simulink model "SIM_Pgrado_Raul"  (R2017a)
settings: Solver=ode45  StartTime=0.0  StopTime=0.2  RelTol=1e-3  EnableMultiTasking=on
undefined symbols (not defined in the file): st_time, st_time3
libraries: fl_lib x50, nesl_utility x19, powerlib_meascontrol x6, dsparch4 x5
settings Model: Creator=erich  LastModifiedBy=erich
settings DataIOCC: LimitDataPoints=on  SaveFormat=StructureWithTime
settings OptimizationCC: LifeSpan=inf
settings DebuggingCC: SFUnexpectedBacktrackingDiag=warning  SFNoUnconditionalDefaultTransitionDiag=warning  SFExecutionAtInitializationDiag=none
settings HardwareCC: ProdBitPerSizeT=32  ProdBitPerPtrDiffT=32  ProdWordSize=32  ProdHWDeviceType=Specified
settings ModelReferenceCC: PropagateSignalLabelsOutOfModel=off
settings GRTTargetCC: TargetLangStandard=C89/C90 (ANSI)
settings ConfigComp: CovMetricSettings=dw  CovHtmlReporting=on  CovSaveCumulativeToWorkspaceVar=on  CovSaveSingleToWorkspaceVar=on  CovExternalEMLEnable=off

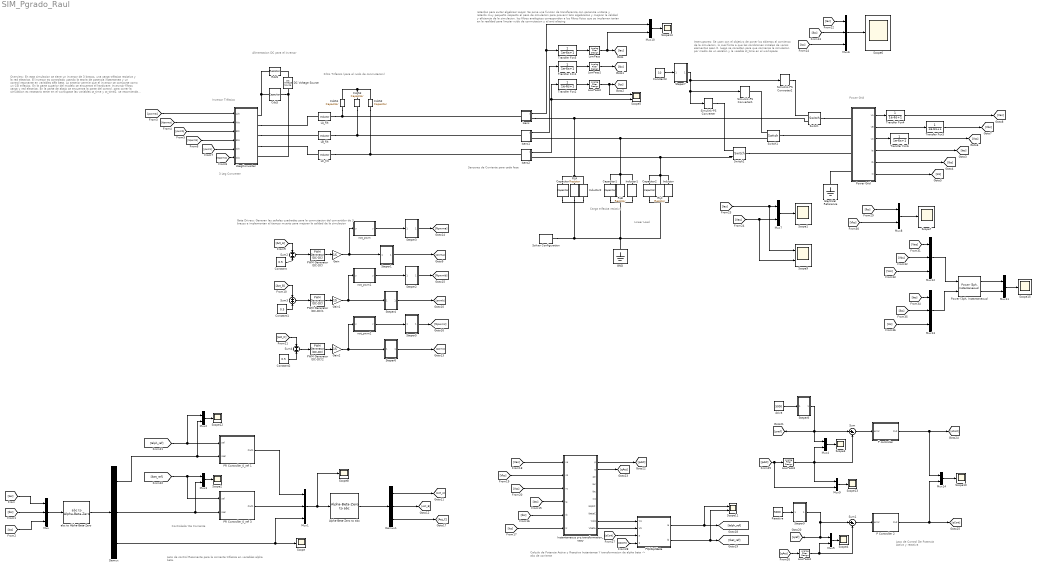
== system SIM_Pgrado_Raul ==
  note: Inversor Trifasico
  note: Overview:
      | En esta simulacion se tiene un inversor
      | de 3 brazos, una carga trifasica resistiva
      | y la red electrica. El inversor es controlado
      | usando la teoria de potencia instantanea
      | y un control resonante en variables alfa beta.
      | Lo anterior permie que el inversor se comporte
      | como un CSI trifasico.
      |
      | En la parte superior del modelo se encuentra el hardware:
      | Invevrsor filtros carga y red electrica.
      |
      | En la parte de abajo se encuentra la parte del control.
      |
      | para correr la simulacion es necesario tener en el workspace
      | las variables st_time y st_time2. se recomienda 10ms y 20 ms
      | respectivamente.
  note: Lazo de Control De
      | Potencia Activa y reactiva
  note: Calculo de Potencia Activa y Reactiva Instantanea
      | Y transformacion de alpha beta -> abc de corriente
  note: retardos para evitar algebraic Loops:
      | Se pone una funcion de transferencia con ganancia unitaria
      | y retardo muy pequeño respecto al paso de simulacion para prevenir
      | lazo algebraicos y mejorar la calidad y eficiencia de la simulacion.
      | los filtros analogicos corresponden a los filtros fisico que se implemen
      | tarian en la realidad para limpiar ruido de conmutacion y el anti aliasing
  note: Power Grid
  note: Linear Load
  note: 3 Leg Converter
  note: Controlador De Corriente
  note: Alimentacion DC
      | para el inversor
  note: Filtro Trifasico
      | (para el ruido de conmutacion)
  note: Sensores de Corriente para cada fase
  note: Carga trifasica resistiva
  note: Interruptores:
      | Se usan con el objetivo de poner
      | los abiertos al comienzo de la simulacion,
      | lo cual forza a que las condiciones iniciales
      | de varios elementos sean 0. luego se conectan
      | para que comience la simulacion por medio de
      | un escalon y la vaiable st_time en el workspace
  note: Lazo de control Resonante para la
      | corriente trifasica en variables alpha beta.
  note: Gate Drivers: Generan las señales cuadradas para
      | la conmutacion del convertidor de 3 brazos e implementan el
      | tiempo muerto para mejorar la calidad de la simulacion
  3LegConverter : Subsystem
  Aciva : Constant  Value=5000
  Alpha-Beta-Zero to abc : powerlib_meascontrol/Transformations/Alpha-Beta-Zero to abc
      settings: SourceProductName=Simscape Power Systems  SourceProductBaseCode=PS
  Capacitor : fl_lib/Electrical/Electrical Elements/Capacitor  c=100e-6 uF  r=1e-6 Ohm  g=0 1/Ohm  i_specify=off  i_priority=None  i=0 A  i_nominal_specify=off  i_nominal_unit=A  i_nominal_value=1  v_specify=off  v_priority=None  v=0 V  v_nominal_specify=off  v_nominal_unit=V  v_nominal_value=1  vc_specify=off  vc_priority=High  vc=0 V  vc_nominal_specify=off  vc_nominal_unit=V  vc_nominal_value=1
  Capacitor1 : fl_lib/Electrical/Electrical Elements/Capacitor  c=100e-6 uF  r=1e-6 Ohm  g=0 1/Ohm  i_specify=off  i_priority=None  i=0 A  i_nominal_specify=off  i_nominal_unit=A  i_nominal_value=1  v_specify=off  v_priority=None  v=0 V  v_nominal_specify=off  v_nominal_unit=V  v_nominal_value=1  vc_specify=off  vc_priority=High  vc=0 V  vc_nominal_specify=off  vc_nominal_unit=V  vc_nominal_value=1
  Capacitor2 : fl_lib/Electrical/Electrical Elements/Capacitor  c=100e-6 uF  r=1e-6 Ohm  g=0 1/Ohm  i_specify=off  i_priority=None  i=0 A  i_nominal_specify=off  i_nominal_unit=A  i_nominal_value=1  v_specify=off  v_priority=None  v=0 V  v_nominal_specify=off  v_nominal_unit=V  v_nominal_value=1  vc_specify=off  vc_priority=High  vc=0 V  vc_nominal_specify=off  vc_nominal_unit=V  vc_nominal_value=1
  CdcS : fl_lib/Electrical/Electrical Elements/Capacitor  c=1 uF  r=1e-6 Ohm  g=0 1/Ohm  i_specify=off  i_priority=None  i=0 A  i_nominal_specify=off  i_nominal_unit=A  i_nominal_value=1  v_specify=off  v_priority=None  v=0 V  v_nominal_specify=off  v_nominal_unit=V  v_nominal_value=1  vc_specify=on  vc_priority=High  vc=0 V  vc_nominal_specify=off  vc_nominal_unit=V  vc_nominal_value=1
  CdcS1 : fl_lib/Electrical/Electrical Elements/Capacitor  c=3.5 uF  r=1e-6 Ohm  g=0 1/Ohm  i_specify=off  i_priority=None  i=0 A  i_nominal_specify=off  i_nominal_unit=A  i_nominal_value=1  v_specify=off  v_priority=None  v=0 V  v_nominal_specify=off  v_nominal_unit=V  v_nominal_value=1  vc_specify=on  vc_priority=High  vc=0 V  vc_nominal_specify=off  vc_nominal_unit=V  vc_nominal_value=1
  CdcS2 : fl_lib/Electrical/Electrical Elements/Capacitor  c=3.5 uF  r=1e-6 Ohm  g=0 1/Ohm  i_specify=off  i_priority=None  i=0 A  i_nominal_specify=off  i_nominal_unit=A  i_nominal_value=1  v_specify=off  v_priority=None  v=0 V  v_nominal_specify=off  v_nominal_unit=V  v_nominal_value=1  vc_specify=on  vc_priority=High  vc=0 V  vc_nominal_specify=off  vc_nominal_unit=V  vc_nominal_value=1
  CdcS3 : fl_lib/Electrical/Electrical Elements/Capacitor  c=3.5 uF  r=1e-6 Ohm  g=0 1/Ohm  i_specify=off  i_priority=None  i=0 A  i_nominal_specify=off  i_nominal_unit=A  i_nominal_value=1  v_specify=off  v_priority=None  v=0 V  v_nominal_specify=off  v_nominal_unit=V  v_nominal_value=1  vc_specify=on  vc_priority=High  vc=0 V  vc_nominal_specify=off  vc_nominal_unit=V  vc_nominal_value=1
  Constant : Constant  Value=0.5
  Constant1 : Constant  Value=0.5
  Constant2 : Constant  Value=0.5
  Constant3 : Constant  Value=10
  DC Voltage Source : fl_lib/Electrical/Electrical Sources/DC Voltage Source  v0=420 V
  Demux : Demux  Outputs=3
  Demux1 : Demux  Outputs=3
  Electrical Reference : fl_lib/Electrical/Electrical Elements/Electrical Reference
  GND : fl_lib/Electrical/Electrical Elements/Electrical Reference
  Gain : Gain  Gain=15
  Gain1 : Gain  Gain=15
  Gain2 : Gain  Gain=15
  Inductor : fl_lib/Electrical/Electrical Elements/Inductor  l=5200 mH  r=0 Ohm  g=100e-9 1/Ohm  i_specify=off  i_priority=None  i=0 A  i_nominal_specify=off  i_nominal_unit=A  i_nominal_value=1  v_specify=off  v_priority=None  v=0 V  v_nominal_specify=off  v_nominal_unit=V  v_nominal_value=1  i_L_specify=off  i_L_priority=High  i_L=0 A  i_L_nominal_specify=off  i_L_nominal_unit=A  i_L_nominal_value=1
  Inductor1 : fl_lib/Electrical/Electrical Elements/Inductor  l=5200 mH  r=0 Ohm  g=100e-9 1/Ohm  i_specify=off  i_priority=None  i=0 A  i_nominal_specify=off  i_nominal_unit=A  i_nominal_value=1  v_specify=off  v_priority=None  v=0 V  v_nominal_specify=off  v_nominal_unit=V  v_nominal_value=1  i_L_specify=off  i_L_priority=High  i_L=0 A  i_L_nominal_specify=off  i_L_nominal_unit=A  i_L_nominal_value=1
  Inductor2 : fl_lib/Electrical/Electrical Elements/Inductor  l=5200 mH  r=0 Ohm  g=100e-9 1/Ohm  i_specify=off  i_priority=None  i=0 A  i_nominal_specify=off  i_nominal_unit=A  i_nominal_value=1  v_specify=off  v_priority=None  v=0 V  v_nominal_specify=off  v_nominal_unit=V  v_nominal_value=1  i_L_specify=off  i_L_priority=High  i_L=0 A  i_L_nominal_specify=off  i_L_nominal_unit=A  i_L_nominal_value=1
  Instantaneous p-q transformation_copy : MATLAB Function  TreatAsAtomicUnit=on
  Isens : Subsystem
  Isens1 : Subsystem
  Isens2 : Subsystem
  LA_filt : fl_lib/Electrical/Electrical Elements/Inductor  l=6.2 mH  r=0.1 Ohm  g=1e-6 1/Ohm  i_specify=off  i_priority=None  i=0 A  i_nominal_specify=off  i_nominal_unit=A  i_nominal_value=1  v_specify=off  v_priority=None  v=0 V  v_nominal_specify=off  v_nominal_unit=V  v_nominal_value=1  i_L_specify=on  i_L_priority=High  i_L=0 A  i_L_nominal_specify=off  i_L_nominal_unit=A  i_L_nominal_value=1
  LB_filt : fl_lib/Electrical/Electrical Elements/Inductor  l=6.2 mH  r=2 Ohm  g=1e-6 1/Ohm  i_specify=off  i_priority=None  i=0 A  i_nominal_specify=off  i_nominal_unit=A  i_nominal_value=1  v_specify=off  v_priority=None  v=0 V  v_nominal_specify=off  v_nominal_unit=V  v_nominal_value=1  i_L_specify=on  i_L_priority=High  i_L=0 A  i_L_nominal_specify=off  i_L_nominal_unit=A  i_L_nominal_value=1
  LC_filt : fl_lib/Electrical/Electrical Elements/Inductor  l=6.2 mH  r=2 Ohm  g=1e-6 1/Ohm  i_specify=off  i_priority=None  i=0 A  i_nominal_specify=off  i_nominal_unit=A  i_nominal_value=1  v_specify=off  v_priority=None  v=0 V  v_nominal_specify=off  v_nominal_unit=V  v_nominal_value=1  i_L_specify=on  i_L_priority=High  i_L=0 A  i_L_nominal_specify=off  i_L_nominal_unit=A  i_L_nominal_value=1
  LowPass{,1..4} (5 alike) : dsparch4/Analog Filter Design  method=Bessel  filttype=Lowpass  N=1  Wlo=2500*2*pi  Whi=80  Rp=2  Rs=40
  Mux{,1,6,12..13} (5 alike) : Mux  Inputs=3
  Mux{2..5,7..11,14} (10 alike) : Mux  Inputs=2
  "P Controller 2 " : Subsystem
  P controller : Subsystem
  PQ2AlphBeta : MATLAB Function  TreatAsAtomicUnit=on
  PR Controller_0_ref 1 : Subsystem
      mask Display:
      | port_label('input',1,'ref')
      | port_label('input',2,'sens')
      | port_label('output',1,'out')
      | 
      | plot(.4+[0:.01:pi/10], .32+sin(40*[0:.01:pi/10])/13)
      | 
      | plot([.4 .6],.05+[.5 .7])
      | plot([.4 .6],.05+[.9 .7])
      | plot([.4 .4],.05+[.9 .5])
      | 
      | text(.27,.37,'\fontsize{25} \int', 'texmode', 'on')
  PR Controller_0_ref 3 : Subsystem
      mask Display:
      | port_label('input',1,'ref')
      | port_label('input',2,'sens')
      | port_label('output',1,'out')
      | 
      | plot(.4+[0:.01:pi/10], .32+sin(40*[0:.01:pi/10])/13)
      | 
      | plot([.4 .6],.05+[.5 .7])
      | plot([.4 .6],.05+[.9 .7])
      | plot([.4 .4],.05+[.9 .5])
      | 
      | text(.27,.37,'\fontsize{25} \int', 'texmode', 'on')
  PWM Generator (DC-DC) : powerlib_meascontrol/Pulse & Signal Generators/PWM Generator (DC-DC)  Fsw=5000  Ts=0
  PWM Generator (DC-DC)1 : powerlib_meascontrol/Pulse & Signal Generators/PWM Generator (DC-DC)  Fsw=5000  Ts=0
  PWM Generator (DC-DC)2 : powerlib_meascontrol/Pulse & Signal Generators/PWM Generator (DC-DC)  Fsw=5000  Ts=0
  "Power (3ph, Instantaneous)" : powerlib_meascontrol/Measurements/Power (3ph, Instantaneous)
      settings: SourceProductName=Simscape Power Systems
  Power Grid : Subsystem
  RLA : fl_lib/Electrical/Electrical Elements/Resistor  R=15 Ohm  i_specify=off  i_priority=None  i=0 A  i_nominal_specify=off  i_nominal_unit=A  i_nominal_value=1  v_specify=off  v_priority=None  v=0 V  v_nominal_specify=off  v_nominal_unit=V  v_nominal_value=1
  RLB : fl_lib/Electrical/Electrical Elements/Resistor  R=15 Ohm  i_specify=off  i_priority=None  i=0 A  i_nominal_specify=off  i_nominal_unit=A  i_nominal_value=1  v_specify=off  v_priority=None  v=0 V  v_nominal_specify=off  v_nominal_unit=V  v_nominal_value=1
  RLC : fl_lib/Electrical/Electrical Elements/Resistor  R=15 Ohm  i_specify=off  i_priority=None  i=0 A  i_nominal_specify=off  i_nominal_unit=A  i_nominal_value=1  v_specify=off  v_priority=None  v=0 V  v_nominal_specify=off  v_nominal_unit=V  v_nominal_value=1
  RdcS : fl_lib/Electrical/Electrical Elements/Resistor  R=0.1 Ohm  i_specify=off  i_priority=None  i=0 A  i_nominal_specify=off  i_nominal_unit=A  i_nominal_value=1  v_specify=off  v_priority=None  v=0 V  v_nominal_specify=off  v_nominal_unit=V  v_nominal_value=1
  Reactiva : Constant  Value=5000
  Scope{,1..4,6..8,10,12..15} (13 alike) : Scope
  Scope11 : Scope  NumInputPorts=2
  Scope5 : Scope  NumInputPorts=2
  Scope9 : Scope  NumInputPorts=2
  Simulink-PS Converter : nesl_utility/Simulink-PS Converter  PhysicalDomain=network_engine_domain  SubClassName=ps_input  LeftPortType=input  RightPortType=output  PseudoPeriodic=off  Frequencies=[]  NoiseDistribution=none  NoiseParameters=[]  Unit=1  AffineConversion=off  FilteringAndDerivatives=zero  SimscapeFilterOrder=1  InputFilterTimeConstant=0.001  UdotUserProvided=1
  Simulink-PS Converter1 : nesl_utility/Simulink-PS Converter  PhysicalDomain=network_engine_domain  SubClassName=ps_input  LeftPortType=input  RightPortType=output  PseudoPeriodic=off  Frequencies=[]  NoiseDistribution=none  NoiseParameters=[]  Unit=1  AffineConversion=off  FilteringAndDerivatives=zero  SimscapeFilterOrder=1  InputFilterTimeConstant=0.001  UdotUserProvided=1
  Simulink-PS Converter2 : nesl_utility/Simulink-PS Converter  PhysicalDomain=network_engine_domain  SubClassName=ps_input  LeftPortType=input  RightPortType=output  PseudoPeriodic=off  Frequencies=[]  NoiseDistribution=none  NoiseParameters=[]  Unit=1  AffineConversion=off  FilteringAndDerivatives=zero  SimscapeFilterOrder=1  InputFilterTimeConstant=0.001  UdotUserProvided=1
  Solver Configuration : nesl_utility/Solver Configuration  PhysicalDomain=network_engine_domain  SubClassName=solver  LeftPortType=input  RightPortType=generic  Accelerate=off  Tones=[]  Harmonics=[]  SimulateNoise=off  Profile=off  UseLocalSampling=off  EnableSwitchedLinearOptims=on  FrequencyDomain=off  UseCCode=off  RelTol=0.001  AbsTol=1e-06  MinStep=1e-09  ToWorkspace=off  RevertToSquareIcSolve=off  NumHomotopyIterations=100  PhasorMode=off  PhasorModeNumHarmonics=1  OverrideAbsTol=off  DoDC=off  ResidualTolerance=1e-09  UseLocalSolver=on  LocalSolverChoice=NE_BACKWARD_EULER_ADVANCER  LocalSolverSampleTime=1e-6  DoFixedCost=on  MaxNonlinIter=3  MaxModeIter=2  LinearAlgebra=Sparse  DelaysMemoryBudget=1024  AutomaticFiltering=on  FilteringTimeConstant=0.001
  Steper1 : Subsystem
  Steper2 : Subsystem
  Steper3 : Subsystem
  Steper4 : Subsystem
  Steper5 : Subsystem
  Steper6 : Subsystem
  Steper7 : Subsystem
  Steper8 : Subsystem
  Steper9 : Subsystem
  Sum : Sum  Inputs=|+-
  Sum1 : Sum  Inputs=|+-
  Sum2 : Sum
  Sum3 : Sum
  Sum4 : Sum
  Switch : fl_lib/Electrical/Electrical Elements/Switch  R_closed=1 Ohm  G_open=1e-4 1/Ohm  Threshold=4  i_specify=off  i_priority=None  i=0 A  i_nominal_specify=off  i_nominal_unit=A  i_nominal_value=1  v_specify=off  v_priority=None  v=0 V  v_nominal_specify=off  v_nominal_unit=V  v_nominal_value=1
      settings: SourceProductName=Simscape
  Switch1 : fl_lib/Electrical/Electrical Elements/Switch  R_closed=1 Ohm  G_open=1e-4 1/Ohm  Threshold=4  i_specify=off  i_priority=None  i=0 A  i_nominal_specify=off  i_nominal_unit=A  i_nominal_value=1  v_specify=off  v_priority=None  v=0 V  v_nominal_specify=off  v_nominal_unit=V  v_nominal_value=1
      settings: SourceProductName=Simscape
  Switch2 : fl_lib/Electrical/Electrical Elements/Switch  R_closed=1 Ohm  G_open=1e-4 1/Ohm  Threshold=4  i_specify=off  i_priority=None  i=0 A  i_nominal_specify=off  i_nominal_unit=A  i_nominal_value=1  v_specify=off  v_priority=None  v=0 V  v_nominal_specify=off  v_nominal_unit=V  v_nominal_value=1
      settings: SourceProductName=Simscape
  Transfer Fcn{1..6} (6 alike) : TransferFcn  Denominator=[1e-6 1]
  abc to Alpha-Beta-Zero : powerlib_meascontrol/Transformations/abc to Alpha-Beta-Zero
      settings: SourceProductName=Simscape Power Systems
  not_pwm : MATLAB Function  TreatAsAtomicUnit=on
  not_pwm1 : MATLAB Function  TreatAsAtomicUnit=on
  not_pwm2 : MATLAB Function  TreatAsAtomicUnit=on
  wires:
  Mux/1 -> abc to Alpha-Beta-Zero/1
  Isens2/1(i) -> Scope5/2, Transfer Fcn2/1
  Isens1/1(i) -> Transfer Fcn1/1
  [Iac] -> Mux/1
  [Ibc] -> Mux/2
  [Icc] -> Mux/3
  abc to Alpha-Beta-Zero/1 -> Demux/1
  Mux1/1 -> Scope8/1, Alpha-Beta-Zero to abc/1
  PR Controller_0_ref 3/1(Out1) -> Mux1/2
  Alpha-Beta-Zero to abc/1 -> Demux1/1
  [pwma] -> 3LegConverter/1(Ahi)
  [Npwmc] -> 3LegConverter/6(Clo)
  [pwmc] -> 3LegConverter/5(Chi)
  [Npwmb] -> 3LegConverter/4(Blo)
  [pwmb] -> 3LegConverter/3(Bhi)
  [Npwma] -> 3LegConverter/2(Alo)
  PWM Generator (DC-DC)/1 -> Gain/1
  PWM Generator (DC-DC)1/1 -> Gain1/1
  PWM Generator (DC-DC)2/1 -> Gain2/1
  not_pwm/1(y) -> Steper3/1(In1)
  not_pwm1/1(y) -> Steper2/1(In1)
  not_pwm2/1(y) -> Steper5/1(In1)
  Gain/1 -> Steper1/1(In1), not_pwm/1(u)
  Gain1/1 -> Steper4/1(In1), not_pwm1/1(u)
  Gain2/1 -> Steper6/1(In1), not_pwm2/1(u)
  Steper3/1(Out1) -> [Npwma]
  Steper2/1(Out1) -> [Npwmb]
  Steper5/1(Out1) -> [Npwmc]
  Steper4/1(Out1) -> [pwmb]
  Steper6/1(Out1) -> [pwmc]
  Transfer Fcn5/1 -> LowPass/1
  Transfer Fcn1/1 -> LowPass1/1
  Transfer Fcn2/1 -> LowPass2/1
  Demux1/1 -> [Act_A]
  Demux1/2 -> [Act_B]
  Demux1/3 -> [Act_C]
  Demux/1 -> PR Controller_0_ref 1/2(real), Mux2/2
  Demux/2 -> PR Controller_0_ref 3/2(real), Mux3/2
  Aciva/1 -> Steper8/1(In1)
  Power Grid/1(vA) -> Transfer Fcn4/1
  Power Grid/2(vB) -> Transfer Fcn3/1
  Power Grid/3(vC) -> Transfer Fcn6/1
  Power Grid/4(Ia) -> [Ias]
  Power Grid/5(Ib) -> [Ibs]
  Power Grid/6(Ic) -> [Ics]
  Reactiva/1 -> Steper9/1(In1)
  [pCont] -> PQ2AlphBeta/3(p)
  [qCont] -> PQ2AlphBeta/4(q)
  P controller/1(Out) -> Mux14/1, [pCont]
  "P Controller 2 "/1(Out) -> Mux14/2, [qCont]
  Constant/1 -> Sum2/2
  Constant1/1 -> Sum3/2
  Constant2/1 -> Sum4/2
  Sum2/1 -> PWM Generator (DC-DC)/1
  [Act_A] -> Sum2/1
  Sum3/1 -> PWM Generator (DC-DC)1/1
  [Act_B] -> Sum3/1
  Sum4/1 -> PWM Generator (DC-DC)2/1
  [Act_C] -> Sum4/1
  Steper7/1(Out1) -> Simulink-PS Converter/1, Simulink-PS Converter1/1, Simulink-PS Converter2/1
  Constant3/1 -> Steper7/1(In1)
  PR Controller_0_ref 1/1(Out1) -> Mux1/1
  Demux/3 -> Mux1/3, Scope/1
  Instantaneous p-q transformation_copy/2(q) -> [qAct]
  Instantaneous p-q transformation_copy/1(p) -> [pAct]
  Instantaneous p-q transformation_copy/10(VbetA) -> PQ2AlphBeta/2(Vb)
  Instantaneous p-q transformation_copy/9(ValA) -> PQ2AlphBeta/1(Va)
  [Iac] -> Instantaneous p-q transformation_copy/4(ia)
  [Ibc] -> Instantaneous p-q transformation_copy/5(ib)
  [Icc] -> Instantaneous p-q transformation_copy/6(ic)
  [Vcs] -> Instantaneous p-q transformation_copy/3(vc)
  [Vbs] -> Instantaneous p-q transformation_copy/2(vb)
  [Vas] -> Instantaneous p-q transformation_copy/1(va)
  Transfer Fcn4/1 -> [Vas]
  Transfer Fcn3/1 -> [Vbs]
  Transfer Fcn6/1 -> [Vcs]
  [Ialph_ref] -> PR Controller_0_ref 1/1(ref), Mux2/1
  [Ibet_ref] -> PR Controller_0_ref 3/1(ref), Mux3/1
  [qAct] -> LowPass4/1
  Sum/1 -> P controller/1(error)
  Sum1/1 -> "P Controller 2 "/1(error)
  Mux2/1 -> Scope12/1
  Mux3/1 -> Scope2/1
  Mux4/1 -> Scope3/1
  Mux5/1 -> Scope4/1
  Mux6/1 -> Scope6/1
  [Iac] -> Mux6/1
  [Ibc] -> Mux6/2
  [Icc] -> Mux6/3
  [Ias] -> Scope9/1, Mux7/1
  Mux7/1 -> Scope1/1
  [Vas] -> Scope9/2, Mux7/2
  Mux8/1 -> Scope7/1
  [Ibs] -> Mux8/1
  [Vbs] -> Mux8/2
  LowPass/1 -> Mux10/2, [Iac]
  LowPass1/1 -> [Ibc]
  LowPass2/1 -> Scope5/1, [Icc]
  Mux9/1 -> Scope13/1
  Mux10/1 -> Scope14/1
  Isens/1(i) -> Transfer Fcn5/1, Mux10/1
  PQ2AlphBeta/1(Ia) -> [Ialph_ref], Scope11/1
  PQ2AlphBeta/2(Ib) -> [Ibet_ref], Scope11/2
  LowPass3/1 -> Mux9/1, Sum/2, Mux4/2
  LowPass4/1 -> Mux5/2, Sum1/2
  [pAct] -> Mux9/2, LowPass3/1
  Mux11/1 -> Scope15/1
  "Power (3ph, Instantaneous)"/1 -> Mux11/1
  "Power (3ph, Instantaneous)"/2 -> Mux11/2
  [Vas] -> Mux12/1
  [Vbs] -> Mux12/2
  [Vcs] -> Mux12/3
  Mux12/1 -> "Power (3ph, Instantaneous)"/1
  [Ias] -> Mux13/1
  [Ibs] -> Mux13/2
  [Ics] -> Mux13/3
  Mux13/1 -> "Power (3ph, Instantaneous)"/2
  Mux14/1 -> Scope10/1
  Steper1/1(Out1) -> [pwma]
  Steper8/1(Out1) -> Mux4/1, Sum/1, [pref]
  Steper9/1(Out1) -> Sum1/1, Mux5/1, [qref]
  connections:
  Power Grid/LConn4 -- Electrical Reference/LConn1
  Isens/RConn1 -- Switch/RConn2 -- Inductor2/LConn1 -- Capacitor/LConn1 -- RLA/LConn1
  RLC/LConn1 -- Capacitor2/LConn1 -- Inductor/LConn1 -- Isens2/RConn1 -- Switch2/RConn2
  RLB/LConn1 -- Capacitor1/LConn1 -- Inductor1/LConn1 -- Isens1/RConn1 -- Switch1/RConn2
  3LegConverter/RConn2 -- LA_filt/LConn1
  3LegConverter/RConn3 -- LB_filt/LConn1
  3LegConverter/RConn4 -- LC_filt/LConn1
  3LegConverter/RConn1 -- RdcS/LConn1 -- CdcS/LConn1
  DC Voltage Source/RConn1 -- CdcS/RConn1 -- 3LegConverter/RConn5
  Solver Configuration/RConn1 -- Inductor2/RConn1 -- Capacitor/RConn1 -- RLA/RConn1 -- Capacitor2/RConn1 -- Inductor/RConn1 -- RLC/RConn1 -- Capacitor1/RConn1 -- Inductor1/RConn1 -- RLB/RConn1 -- GND/LConn1
  DC Voltage Source/LConn1 -- RdcS/RConn1
  Switch/LConn1 -- Power Grid/LConn1
  Switch1/LConn1 -- Power Grid/LConn2
  Switch2/LConn1 -- Power Grid/LConn3
  Switch1/RConn1 -- Simulink-PS Converter1/RConn1
  Simulink-PS Converter2/RConn1 -- Switch/RConn1
  Simulink-PS Converter/RConn1 -- Switch2/RConn1
  LA_filt/RConn1 -- Isens/LConn1 -- CdcS1/RConn1
  LB_filt/RConn1 -- Isens1/LConn1 -- CdcS3/RConn1
  LC_filt/RConn1 -- Isens2/LConn1 -- CdcS2/RConn1
  CdcS1/LConn1 -- CdcS3/LConn1 -- CdcS2/LConn1

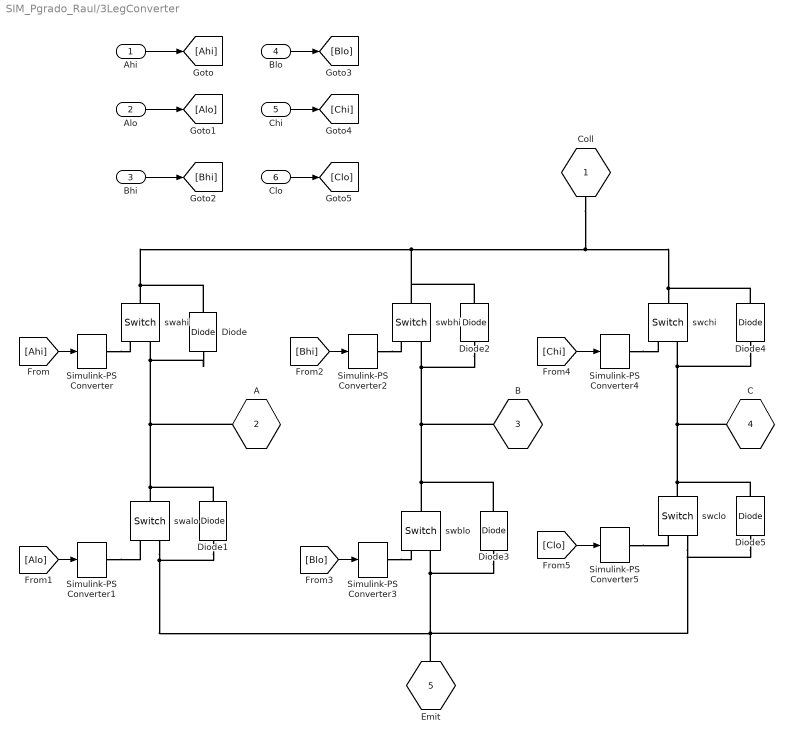
== system SIM_Pgrado_Raul/3LegConverter ==
  Ahi : Inport
  Alo : Inport  Port=2
  Bhi : Inport  Port=3
  Blo : Inport  Port=4
  Chi : Inport  Port=5
  Clo : Inport  Port=6
  Diode{,1..5} (6 alike) : fl_lib/Electrical/Electrical Elements/Diode  Vf=0.6 V  Ron=0.3 Ohm  Goff=1e-8 1/Ohm  i_specify=off  i_priority=None  i=0 A  i_nominal_specify=off  i_nominal_unit=A  i_nominal_value=1  v_specify=off  v_priority=None  v=0 V  v_nominal_specify=off  v_nominal_unit=V  v_nominal_value=1
  Simulink-PS Converter{,1..5} (6 alike) : nesl_utility/Simulink-PS Converter  PhysicalDomain=network_engine_domain  SubClassName=ps_input  LeftPortType=input  RightPortType=output  PseudoPeriodic=off  Frequencies=[]  NoiseDistribution=none  NoiseParameters=[]  Unit=1  AffineConversion=off  FilteringAndDerivatives=zero  SimscapeFilterOrder=1  InputFilterTimeConstant=0.001  UdotUserProvided=1
  swahi : fl_lib/Electrical/Electrical Elements/Switch  R_closed=0.01 Ohm  G_open=1e-8 1/Ohm  Threshold=2  i_specify=off  i_priority=None  i=0 A  i_nominal_specify=off  i_nominal_unit=A  i_nominal_value=1  v_specify=off  v_priority=None  v=0 V  v_nominal_specify=off  v_nominal_unit=V  v_nominal_value=1
      settings: SourceProductName=Simscape
  swalo : fl_lib/Electrical/Electrical Elements/Switch  R_closed=0.01 Ohm  G_open=1e-8 1/Ohm  Threshold=2  i_specify=off  i_priority=None  i=0 A  i_nominal_specify=off  i_nominal_unit=A  i_nominal_value=1  v_specify=off  v_priority=None  v=0 V  v_nominal_specify=off  v_nominal_unit=V  v_nominal_value=1
      settings: SourceProductName=Simscape
  swbhi : fl_lib/Electrical/Electrical Elements/Switch  R_closed=0.01 Ohm  G_open=1e-8 1/Ohm  Threshold=2  i_specify=off  i_priority=None  i=0 A  i_nominal_specify=off  i_nominal_unit=A  i_nominal_value=1  v_specify=off  v_priority=None  v=0 V  v_nominal_specify=off  v_nominal_unit=V  v_nominal_value=1
      settings: SourceProductName=Simscape
  swblo : fl_lib/Electrical/Electrical Elements/Switch  R_closed=0.01 Ohm  G_open=1e-8 1/Ohm  Threshold=2  i_specify=off  i_priority=None  i=0 A  i_nominal_specify=off  i_nominal_unit=A  i_nominal_value=1  v_specify=off  v_priority=None  v=0 V  v_nominal_specify=off  v_nominal_unit=V  v_nominal_value=1
      settings: SourceProductName=Simscape
  swchi : fl_lib/Electrical/Electrical Elements/Switch  R_closed=0.01 Ohm  G_open=1e-8 1/Ohm  Threshold=2  i_specify=off  i_priority=None  i=0 A  i_nominal_specify=off  i_nominal_unit=A  i_nominal_value=1  v_specify=off  v_priority=None  v=0 V  v_nominal_specify=off  v_nominal_unit=V  v_nominal_value=1
      settings: SourceProductName=Simscape
  swclo : fl_lib/Electrical/Electrical Elements/Switch  R_closed=0.01 Ohm  G_open=1e-8 1/Ohm  Threshold=2  i_specify=off  i_priority=None  i=0 A  i_nominal_specify=off  i_nominal_unit=A  i_nominal_value=1  v_specify=off  v_priority=None  v=0 V  v_nominal_specify=off  v_nominal_unit=V  v_nominal_value=1
      settings: SourceProductName=Simscape
  Coll : PMIOPort  Port=1  Side=Right
  A : PMIOPort  Port=2  Side=Right
  B : PMIOPort  Port=3  Side=Right
  C : PMIOPort  Port=4  Side=Right
  Emit : PMIOPort  Port=5  Side=Right
  wires:
  [Alo] -> Simulink-PS Converter1/1
  [Ahi] -> Simulink-PS Converter/1
  Clo/1 -> [Clo]
  Alo/1 -> [Alo]
  [Blo] -> Simulink-PS Converter3/1
  [Clo] -> Simulink-PS Converter5/1
  Bhi/1 -> [Bhi]
  [Bhi] -> Simulink-PS Converter2/1
  Ahi/1 -> [Ahi]
  [Chi] -> Simulink-PS Converter4/1
  Blo/1 -> [Blo]
  Chi/1 -> [Chi]
  connections:
  swalo/RConn2 -- Diode3/LConn1 -- swblo/RConn2 -- Emit/RConn1 -- Diode5/LConn1 -- swclo/RConn2 -- Diode1/LConn1
  Simulink-PS Converter4/RConn1 -- swchi/RConn1
  Simulink-PS Converter5/RConn1 -- swclo/RConn1
  Simulink-PS Converter/RConn1 -- swahi/RConn1
  swblo/LConn1 -- Diode3/RConn1 -- B/RConn1 -- Diode2/LConn1 -- swbhi/RConn2
  Simulink-PS Converter3/RConn1 -- swblo/RConn1
  Simulink-PS Converter2/RConn1 -- swbhi/RConn1
  Simulink-PS Converter1/RConn1 -- swalo/RConn1
  swalo/LConn1 -- A/RConn1 -- Diode/LConn1 -- swahi/RConn2 -- Diode1/RConn1
  swahi/LConn1 -- Diode/RConn1 -- Diode2/RConn1 -- swbhi/LConn1 -- Coll/RConn1 -- Diode4/RConn1 -- swchi/LConn1
  swclo/LConn1 -- Diode5/RConn1 -- C/RConn1 -- Diode4/LConn1 -- swchi/RConn2

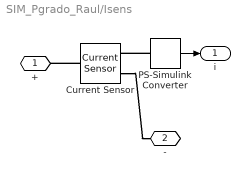
== system SIM_Pgrado_Raul/Isens ==
  Current Sensor : fl_lib/Electrical/Electrical Sensors/Current Sensor
  PS-Simulink Converter : nesl_utility/PS-Simulink Converter  PhysicalDomain=network_engine_domain  SubClassName=ps_output  LeftPortType=input  RightPortType=output  PseudoPeriodic=off  Frequencies=[]  Unit=1  AffineConversion=off
  + : PMIOPort  Port=1  Side=Left
  - : PMIOPort  Port=2  Side=Right
  i : Outport
  wires:
  PS-Simulink Converter/1 -> i/1
  connections:
  PS-Simulink Converter/LConn1 -- Current Sensor/RConn1
  Current Sensor/RConn2 -- -/RConn1
  Current Sensor/LConn1 -- +/RConn1

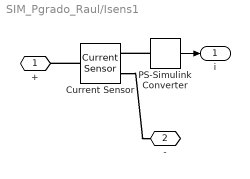
== system SIM_Pgrado_Raul/Isens1 ==
  Current Sensor : fl_lib/Electrical/Electrical Sensors/Current Sensor
  PS-Simulink Converter : nesl_utility/PS-Simulink Converter  PhysicalDomain=network_engine_domain  SubClassName=ps_output  LeftPortType=input  RightPortType=output  PseudoPeriodic=off  Frequencies=[]  Unit=1  AffineConversion=off
  + : PMIOPort  Port=1  Side=Left
  - : PMIOPort  Port=2  Side=Right
  i : Outport
  wires:
  PS-Simulink Converter/1 -> i/1
  connections:
  Current Sensor/LConn1 -- +/RConn1
  Current Sensor/RConn2 -- -/RConn1
  PS-Simulink Converter/LConn1 -- Current Sensor/RConn1

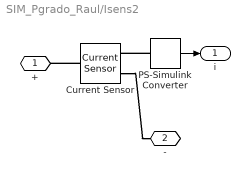
== system SIM_Pgrado_Raul/Isens2 ==
  Current Sensor : fl_lib/Electrical/Electrical Sensors/Current Sensor
  PS-Simulink Converter : nesl_utility/PS-Simulink Converter  PhysicalDomain=network_engine_domain  SubClassName=ps_output  LeftPortType=input  RightPortType=output  PseudoPeriodic=off  Frequencies=[]  Unit=1  AffineConversion=off
  + : PMIOPort  Port=1  Side=Left
  - : PMIOPort  Port=2  Side=Right
  i : Outport
  wires:
  PS-Simulink Converter/1 -> i/1
  connections:
  PS-Simulink Converter/LConn1 -- Current Sensor/RConn1
  Current Sensor/RConn2 -- -/RConn1
  Current Sensor/LConn1 -- +/RConn1

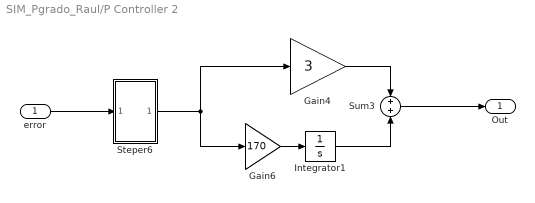
== system SIM_Pgrado_Raul/P Controller 2  ==
  error : Inport
  Gain4 : Gain  Gain=3
  Gain6 : Gain  Gain=170
  Integrator1 : Integrator
  Steper6 : Subsystem
  Sum3 : Sum  Inputs=+|+
  Out : Outport
  wires:
  Gain6/1 -> Integrator1/1
  Gain4/1 -> Sum3/1
  Sum3/1 -> Out/1
  Integrator1/1 -> Sum3/2
  error/1 -> Steper6/1(In1)
  Steper6/1(Out1) -> Gain4/1, Gain6/1

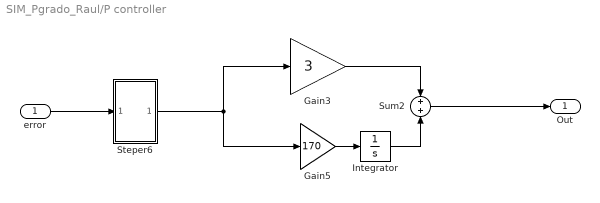
== system SIM_Pgrado_Raul/P controller ==
  error : Inport
  Gain3 : Gain  Gain=3
  Gain5 : Gain  Gain=170
  Integrator : Integrator
  Steper6 : Subsystem
  Sum2 : Sum  Inputs=+|+
  Out : Outport
  wires:
  Gain3/1 -> Sum2/1
  Integrator/1 -> Sum2/2
  Gain5/1 -> Integrator/1
  Sum2/1 -> Out/1
  error/1 -> Steper6/1(In1)
  Steper6/1(Out1) -> Gain5/1, Gain3/1

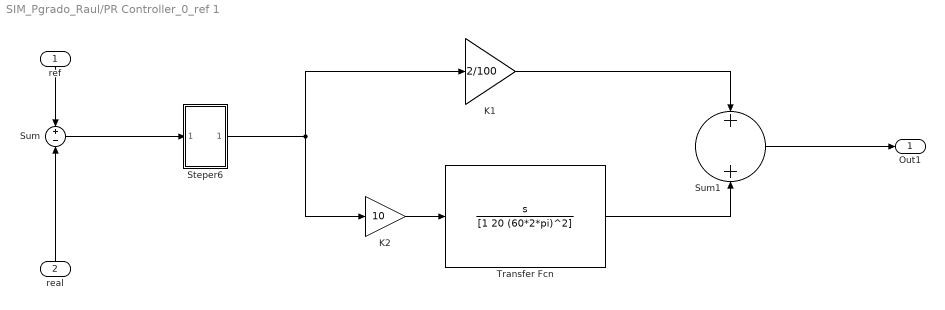
== system SIM_Pgrado_Raul/PR Controller_0_ref 1 ==
  ref : Inport
  real : Inport  Port=2
  K1 : Gain  Gain=2/100
  K2 : Gain  Gain=10
  Steper6 : Subsystem
  Sum : Sum  Inputs=+-
  Sum1 : Sum  Inputs=+|+
  Transfer Fcn : TransferFcn  Numerator=[1 0]  Denominator=[1 20 (60*2*pi)^2]
  Out1 : Outport
  wires:
  Sum1/1 -> Out1/1
  Steper6/1(Out1) -> K2/1, K1/1
  K2/1 -> Transfer Fcn/1
  Transfer Fcn/1 -> Sum1/2
  K1/1 -> Sum1/1
  Sum/1 -> Steper6/1(In1)
  ref/1 -> Sum/1
  real/1 -> Sum/2

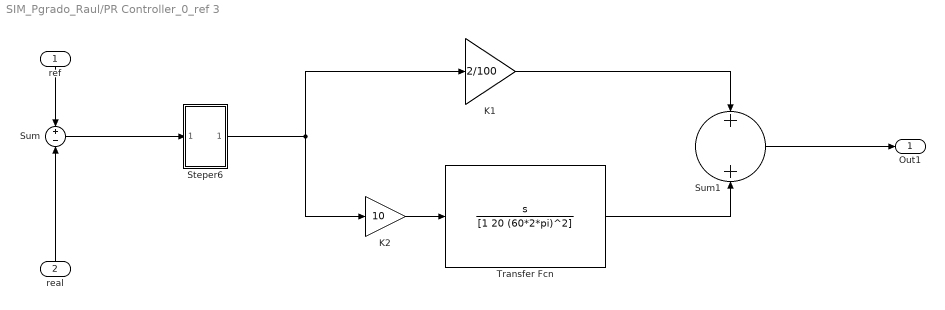
== system SIM_Pgrado_Raul/PR Controller_0_ref 3 ==
  ref : Inport
  real : Inport  Port=2
  K1 : Gain  Gain=2/100
  K2 : Gain  Gain=10
  Steper6 : Subsystem
  Sum : Sum  Inputs=+-
  Sum1 : Sum  Inputs=+|+
  Transfer Fcn : TransferFcn  Numerator=[1 0]  Denominator=[1 20 (60*2*pi)^2]
  Out1 : Outport
  wires:
  real/1 -> Sum/2
  ref/1 -> Sum/1
  Sum/1 -> Steper6/1(In1)
  K1/1 -> Sum1/1
  Transfer Fcn/1 -> Sum1/2
  K2/1 -> Transfer Fcn/1
  Steper6/1(Out1) -> K1/1, K2/1
  Sum1/1 -> Out1/1

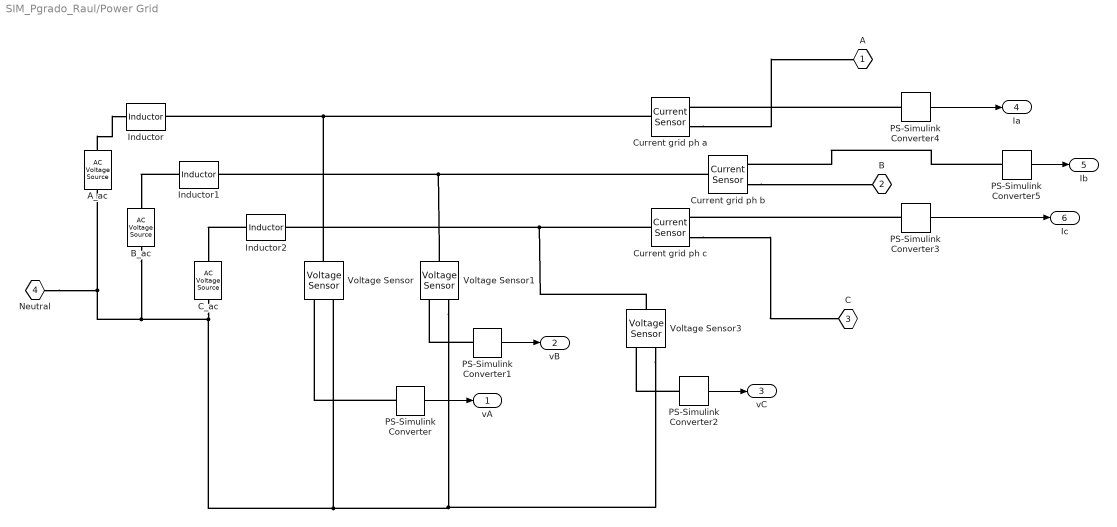
== system SIM_Pgrado_Raul/Power Grid ==
  A_ac : fl_lib/Electrical/Electrical Sources/AC Voltage Source  amp=170 V  shift=0 deg  frequency=60 Hz  omega=0 rad/s
  B_ac : fl_lib/Electrical/Electrical Sources/AC Voltage Source  amp=170 V  shift=-120 deg  frequency=60 Hz  omega=0 rad/s
  C_ac : fl_lib/Electrical/Electrical Sources/AC Voltage Source  amp=170 V  shift=120 deg  frequency=60 Hz  omega=0 rad/s
  Current grid ph a : fl_lib/Electrical/Electrical Sensors/Current Sensor
  Current grid ph b : fl_lib/Electrical/Electrical Sensors/Current Sensor
  Current grid ph c : fl_lib/Electrical/Electrical Sensors/Current Sensor
  Inductor : fl_lib/Electrical/Electrical Elements/Inductor  l=0.1 uH  r=0.2 Ohm  g=1e-9 1/Ohm  i_specify=off  i_priority=None  i=0 A  i_nominal_specify=off  i_nominal_unit=A  i_nominal_value=1  v_specify=off  v_priority=None  v=0 V  v_nominal_specify=off  v_nominal_unit=V  v_nominal_value=1  i_L_specify=on  i_L_priority=High  i_L=0 A  i_L_nominal_specify=off  i_L_nominal_unit=A  i_L_nominal_value=1
  Inductor1 : fl_lib/Electrical/Electrical Elements/Inductor  l=0.1 uH  r=0.2 Ohm  g=1e-9 1/Ohm  i_specify=off  i_priority=None  i=0 A  i_nominal_specify=off  i_nominal_unit=A  i_nominal_value=1  v_specify=off  v_priority=None  v=0 V  v_nominal_specify=off  v_nominal_unit=V  v_nominal_value=1  i_L_specify=on  i_L_priority=High  i_L=0 A  i_L_nominal_specify=off  i_L_nominal_unit=A  i_L_nominal_value=1
  Inductor2 : fl_lib/Electrical/Electrical Elements/Inductor  l=0.1 uH  r=0.2 Ohm  g=1e-9 1/Ohm  i_specify=off  i_priority=None  i=0 A  i_nominal_specify=off  i_nominal_unit=A  i_nominal_value=1  v_specify=off  v_priority=None  v=0 V  v_nominal_specify=off  v_nominal_unit=V  v_nominal_value=1  i_L_specify=on  i_L_priority=High  i_L=0 A  i_L_nominal_specify=off  i_L_nominal_unit=A  i_L_nominal_value=1
  PS-Simulink Converter{,1..5} (6 alike) : nesl_utility/PS-Simulink Converter  PhysicalDomain=network_engine_domain  SubClassName=ps_output  LeftPortType=input  RightPortType=output  PseudoPeriodic=off  Frequencies=[]  Unit=1  AffineConversion=off
  Voltage Sensor : fl_lib/Electrical/Electrical Sensors/Voltage Sensor
  Voltage Sensor1 : fl_lib/Electrical/Electrical Sensors/Voltage Sensor
  Voltage Sensor3 : fl_lib/Electrical/Electrical Sensors/Voltage Sensor
  A : PMIOPort  Port=1  Side=Left
  B : PMIOPort  Port=2  Side=Left
  C : PMIOPort  Port=3  Side=Left
  Neutral : PMIOPort  Port=4  Side=Left
  vA : Outport
  vB : Outport  Port=2
  vC : Outport  Port=3
  Ia : Outport  Port=4
  Ib : Outport  Port=5
  Ic : Outport  Port=6
  wires:
  PS-Simulink Converter/1 -> vA/1
  PS-Simulink Converter1/1 -> vB/1
  PS-Simulink Converter2/1 -> vC/1
  PS-Simulink Converter4/1 -> Ia/1
  PS-Simulink Converter5/1 -> Ib/1
  PS-Simulink Converter3/1 -> Ic/1
  connections:
  Inductor2/LConn1 -- C_ac/LConn1
  A_ac/LConn1 -- Inductor/LConn1
  Inductor1/LConn1 -- B_ac/LConn1
  Voltage Sensor1/LConn1 -- Inductor1/RConn1 -- Current grid ph b/LConn1
  PS-Simulink Converter/LConn1 -- Voltage Sensor/RConn1
  Voltage Sensor3/LConn1 -- Inductor2/RConn1 -- Current grid ph c/LConn1
  Voltage Sensor/LConn1 -- Current grid ph a/LConn1 -- Inductor/RConn1
  A_ac/RConn1 -- Neutral/RConn1 -- Voltage Sensor3/RConn2 -- Voltage Sensor1/RConn2 -- Voltage Sensor/RConn2 -- C_ac/RConn1 -- B_ac/RConn1
  PS-Simulink Converter1/LConn1 -- Voltage Sensor1/RConn1
  PS-Simulink Converter2/LConn1 -- Voltage Sensor3/RConn1
  Current grid ph c/RConn2 -- C/RConn1
  Current grid ph b/RConn2 -- B/RConn1
  Current grid ph a/RConn2 -- A/RConn1
  PS-Simulink Converter3/LConn1 -- Current grid ph c/RConn1
  PS-Simulink Converter4/LConn1 -- Current grid ph a/RConn1
  PS-Simulink Converter5/LConn1 -- Current grid ph b/RConn1

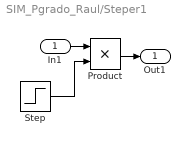
== system SIM_Pgrado_Raul/Steper1 ==
  In1 : Inport
  Product : Product
  Step : Step  Time=st_time3  SampleTime=0
  Out1 : Outport
  wires:
  Step/1 -> Product/2
  In1/1 -> Product/1
  Product/1 -> Out1/1

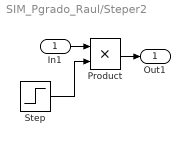
== system SIM_Pgrado_Raul/Steper2 ==
  In1 : Inport
  Product : Product
  Step : Step  Time=st_time3  SampleTime=0
  Out1 : Outport
  wires:
  Product/1 -> Out1/1
  In1/1 -> Product/1
  Step/1 -> Product/2

== system SIM_Pgrado_Raul/Steper3 ==
  In1 : Inport
  Product : Product
  Step : Step  Time=st_time3  SampleTime=0
  Out1 : Outport
  wires:
  Product/1 -> Out1/1
  In1/1 -> Product/1
  Step/1 -> Product/2

== system SIM_Pgrado_Raul/Steper4 ==
  In1 : Inport
  Product : Product
  Step : Step  Time=st_time3  SampleTime=0
  Out1 : Outport
  wires:
  Step/1 -> Product/2
  In1/1 -> Product/1
  Product/1 -> Out1/1

== system SIM_Pgrado_Raul/Steper5 ==
  In1 : Inport
  Product : Product
  Step : Step  Time=st_time3  SampleTime=0
  Out1 : Outport
  wires:
  Product/1 -> Out1/1
  In1/1 -> Product/1
  Step/1 -> Product/2

== system SIM_Pgrado_Raul/Steper6 ==
  In1 : Inport
  Product : Product
  Step : Step  Time=st_time3  SampleTime=0
  Out1 : Outport
  wires:
  Step/1 -> Product/2
  In1/1 -> Product/1
  Product/1 -> Out1/1

== system SIM_Pgrado_Raul/Steper7 ==
  In1 : Inport
  Product : Product
  Step : Step  Time=st_time  SampleTime=0
  Out1 : Outport
  wires:
  Product/1 -> Out1/1
  In1/1 -> Product/1
  Step/1 -> Product/2

== system SIM_Pgrado_Raul/Steper8 ==
  In1 : Inport
  Product : Product
  Step : Step  Time=st_time3  SampleTime=0
  Out1 : Outport
  wires:
  Product/1 -> Out1/1
  In1/1 -> Product/1
  Step/1 -> Product/2

== system SIM_Pgrado_Raul/Steper9 ==
  In1 : Inport
  Product : Product
  Step : Step  Time=st_time3  SampleTime=0
  Out1 : Outport
  wires:
  Product/1 -> Out1/1
  In1/1 -> Product/1
  Step/1 -> Product/2

== system SIM_Pgrado_Raul/P Controller 2 /Steper6 ==
  In1 : Inport
  Product : Product
  Step : Step  Time=st_time3  SampleTime=0
  Out1 : Outport
  wires:
  Product/1 -> Out1/1
  In1/1 -> Product/1
  Step/1 -> Product/2

== system SIM_Pgrado_Raul/P controller/Steper6 ==
  In1 : Inport
  Product : Product
  Step : Step  Time=st_time3  SampleTime=0
  Out1 : Outport
  wires:
  Product/1 -> Out1/1
  In1/1 -> Product/1
  Step/1 -> Product/2

== system SIM_Pgrado_Raul/PR Controller_0_ref 1/Steper6 ==
  In1 : Inport
  Product : Product
  Step : Step  Time=st_time3  SampleTime=0
  Out1 : Outport
  wires:
  Step/1 -> Product/2
  In1/1 -> Product/1
  Product/1 -> Out1/1

== system SIM_Pgrado_Raul/PR Controller_0_ref 3/Steper6 ==
  In1 : Inport
  Product : Product
  Step : Step  Time=st_time3  SampleTime=0
  Out1 : Outport
  wires:
  Product/1 -> Out1/1
  In1/1 -> Product/1
  Step/1 -> Product/2

== matlab function SIM_Pgrado_Raul/not_pwm1 ==
  data: u input; y output
function y = fcn(u)
%#codegen

if(u==0 || u<0)
    a=5;
else
    a=0;
end;

y = a;

== matlab function SIM_Pgrado_Raul/not_pwm ==
  data: u input; y output
function y = fcn(u)
%#codegen

if(u==0 || u<0)
    a=15;
else
    a=0;
end;

y = a;

== matlab function SIM_Pgrado_Raul/not_pwm2 ==
  data: u input; y output
function y = fcn(u)
%#codegen

if(u==0 || u<0)
    a=5;
else
    a=0;
end;

y = a;

== matlab function SIM_Pgrado_Raul/Instantaneous p-q transformation_copy ==
  data: va input; p output; vb input; vc input; ia input; ib input; ic input; q output; p0 output; iac output; ibc output; icc output; ialphC output; ibetaC output; ValA output; VbetA output
function [p, q, p0, iac, ibc, icc, ialphC, ibetaC, ValA, VbetA] = fcn(va, vb, vc, ia, ib, ic)
% Esta funcion calcula la potencia activa y reactiva instantanea
% dados 3 tensiones y 3 corrientes instantaneas.
% para esto se usa version de la transformada de clarke cuya potencia es 
% invariante (power invariant clarke transform).


pi_clarke = [[1 -1/2 -1/2]; [0 sqrt(3)/2 -sqrt(3)/2]; [1/sqrt(2) 1/sqrt(2) 1/sqrt(2)]]*sqrt(2/3);%matriz de clarke

tv = pi_clarke*[va;vb;vc];% transformada de las tensiones
ti = pi_clarke*[ia;ib;ic];%trasnformada de las corrientes

valph = tv(1);% se separa los valores de las transformadas de tension
vbet = tv(2);
v0 = tv(3);

ValA = valph;
VbetA = vbet;

ialph = ti(1);% se separa los valores de la transformda de corriente
ibet = ti(2);
i0 = ti(3);

paux=valph*ialph+vbet*ibet;
if(paux > 20e4)
    paux=20e4;
end;
if(paux < -20e4)
    paux = -20e-4;
end;

p = paux; % potencia activa instantanea

qaux=vbet*ialph-valph*ibet;

if(qaux>20e4)
    qaux=20e4;
end;
if(qaux<-20e4)
    qaux=-20e4;
end;
q = qaux; % potencia reactiva instantanea


p0 = v0*i0; % potencia instantanea de secuencia 0.



mat2cur = [valph vbet; vbet valph]; % matriz para pasar de potencia
% a corrientes por medio de una matriz de tensiones en alpha beta.

det = 1/(valph^2+vbet^2); % constante auxiliar
if(abs(det)<=100*eps(0))
    det=10*eps(0);
end;

mat2cur = mat2cur*det; % matriz final para pasar a corrientes



IabetC = mat2cur*[0; -q]; % vector corriente de compensacion en alpha beta

%inv_clarke = inv([[1 -1/2 -1/2]; [0 sqrt(3)/2 -sqrt(3)/2]; [1/sqrt(2) 1/sqrt(2) 1/sqrt(2)]]*sqrt(2/3));%matriz de clarke

ialphCaux = IabetC(1);
ibetaCaux = IabetC(2);

ilim=10e3;

if(ialphCaux>ilim)
    ialphCaux=ilim;
end;
if(ialphCaux<-ilim)
    ialphCaux =-ilim;    
end;
if(isnan(ialphCaux))
    ialphCaux=0;
end;
%---------------------
if(ibetaCaux>ilim)
    ibetaCaux=ilim;
end;
if(ibetaCaux<-ilim)
    ibetaCaux=-ilim;    
end;
if(isnan(ibetaCaux))
    ibetaCaux=0;
end;
ialphC = ialphCaux;
ibetaC = ibetaCaux;


Icom = pi_clarke\[IabetC(1); IabetC(2); 0];

iacaux = Icom(1);
ibcaux = Icom(2);
iccaux = Icom(3);

if(iacaux>ilim)
    iacaux=ilim;
end;
if(iacaux<-ilim)
    iacaux =-ilim;    
end;
if(isnan(iacaux))
    iacaux=0;
end;
%---------------------
if(ibcaux>ilim)
    ibcaux=ilim;
end;
if(ibcaux<-ilim)
    ibcaux =-ilim;    
end;

if(isnan(ibcaux))
    ibcaux=0;
end;
%-------------
if(iccaux>ilim)
    iccaux=ilim;
end;
if(iccaux<-ilim)
    iccaux =-ilim;    
end;

if(isnan(iccaux))
    iccaux=0;
end;
%-----------------
iac = iacaux;
ibc = ibcaux;
icc = iccaux;

== matlab function SIM_Pgrado_Raul/PQ2AlphBeta ==
  data: Va input; Ia output; Vb input; p input; q input; Ib output
function [Ia, Ib] = fcn(Va, Vb, p, q)
%#codegen

% divide by zero protection
if(abs((Va^2+Vb^2))<=1000*eps(0))
    det = 1/eps(0);
else
    det = 1/(Va^2+Vb^2); % constante auxiliar
end;
%det = 1/(Va^2+Vb^2);

Mat = det*[Va Vb; Vb -Va];
Iab = Mat*[p;q];

Iaaux = Iab(1);
Ibaux = Iab(2);

ilim=1e3;

if(Iaaux>ilim)
    Iaaux=ilim;
end;
if(Iaaux<-ilim)
    Iaaux =-ilim;    
end;

if(isnan(Iaaux))
    Iaaux=0;
end;
%-----------------


if(Ibaux>ilim)
    Ibaux=ilim;
end;
if(Ibaux<-ilim)
    Ibaux =-ilim;    
end;

if(isnan(Ibaux))
    Ibaux=0;
end;
%-----------------


Ia = Iaaux;
Ib = Ibaux;
